simulink model "LQR_nonlinearized"  (R2019a)
settings: Solver=VariableStepAuto  StartTime=0.0  StopTime=10.0  RelTol=1e-3
values from neighbouring files (symbols this model uses):
  A = [0, 0, 1, 0 ... (first row only)    [LQR_v1.m]
  B = [0; 0; 0; b41]    [LQR_v1.m]
  C = [1, 0, 0, 0 ... (first row only)    [LQR_v1.m]
  g = 9.81    [LQR_v1.m]
  hb = 0.37    [LQR_v1.m]
  Igz = 0.061    [LQR_v1.m]
  Init_cond = [roll_angel, precession_angle, roll_rate, precession_rate]    [LQR_v1.m]
  init_precession_angle = 0    [LQR_v1.m]
  init_precession_rate = 0    [LQR_v1.m]
  init_roll_angle = 0.34    [LQR_v1.m]
  init_roll_rate = 0    [LQR_v1.m]
  K = lqr( A, B, Q, R )    [LQR_v1.m]
  k1 = 2*( Icx + Igx )    (= 0.141)    [LQR_v1.m]
  k2 = 2*( Icy + Igy )    (= 0.181)    [LQR_v1.m]
  k3 = 2*( Icz + Igz )    (= 0.322)    [LQR_v1.m]
  k4 = Ibx + 2*Igbx + 2*Isx    (= 10.2)    [LQR_v1.m]
  k5 = k1 - k3    (= -0.181)    [LQR_v1.m]
  k6 = hb*mb + 2*hg*(mg + mc + mgb) + 2*hs*ms    (= 26.27)    [LQR_v1.m]
  k7 = ( hb^2 )*mb + 2*( hg^2 )*( mg + mc + mgb ) + 2*( hs^2 )*ms    (= 9.7199)    [LQR_v1.m]
  omega = 532.6    [LQR_v1.m]
settings Model: Creator=daniel  LastModifiedBy=nata9
settings DataIOCC: ReturnWorkspaceOutputs=off
settings DebuggingCC: ArithmeticOperatorsInVariantConditions=warning
settings SFSimCC: SimUseLocalCustomCode=off
settings RTWCC: RTWUseLocalCustomCode=off

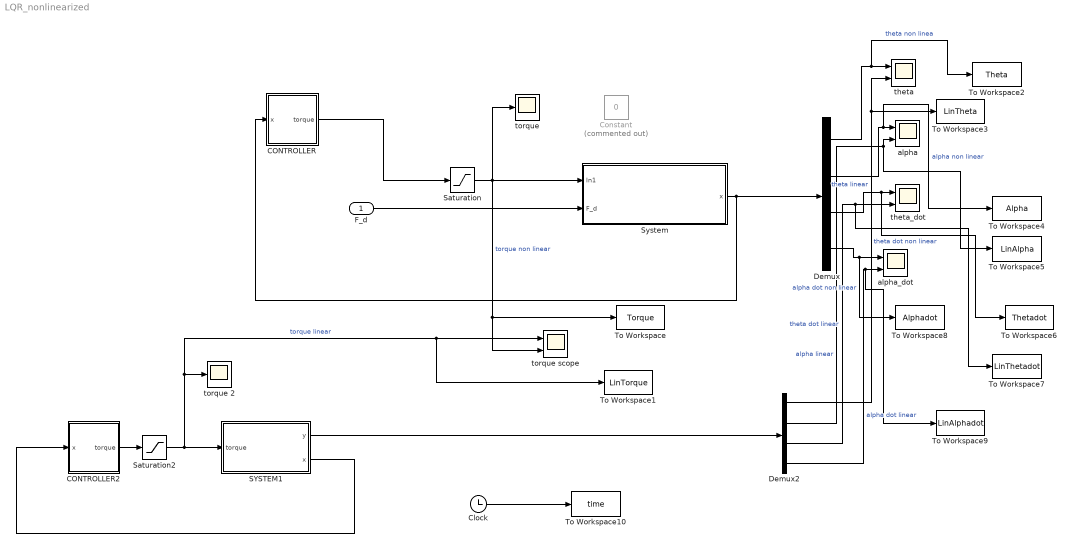
== system LQR_nonlinearized ==
  F_d : Inport
  " System" : Subsystem
  CONTROLLER : Subsystem
  CONTROLLER2 : Subsystem
  Clock : Clock
  Constant : Constant  Commented=on  Value=0
  Demux : Demux
  Demux2 : Demux
  SYSTEM1 : Subsystem
  Saturation : Saturate  UpperLimit=120  LowerLimit=-120
  Saturation2 : Saturate  UpperLimit=120  LowerLimit=-120
  To Workspace : ToWorkspace  VariableName=Torque  SampleTime=-1
  To Workspace1 : ToWorkspace  VariableName=LinTorque  SampleTime=-1
  To Workspace10 : ToWorkspace  VariableName=time  SampleTime=-1
  To Workspace2 : ToWorkspace  VariableName=Theta  SampleTime=-1
  To Workspace3 : ToWorkspace  VariableName=LinTheta  SampleTime=-1
  To Workspace4 : ToWorkspace  VariableName=Alpha  SampleTime=-1
  To Workspace5 : ToWorkspace  VariableName=LinAlpha  SampleTime=-1
  To Workspace6 : ToWorkspace  VariableName=Thetadot  SampleTime=-1
  To Workspace7 : ToWorkspace  VariableName=LinThetadot  SampleTime=-1
  To Workspace8 : ToWorkspace  VariableName=Alphadot  SampleTime=-1
  To Workspace9 : ToWorkspace  VariableName=LinAlphadot  SampleTime=-1
  alpha : Scope  NumInputPorts=2
  alpha_dot : Scope  NumInputPorts=2
  theta : Scope  NumInputPorts=2
  theta_dot : Scope  NumInputPorts=2
  "torque " : Scope
  torque 2 : Scope
  torque scope : Scope  NumInputPorts=2
  wires:
  CONTROLLER/1(torque) -> Saturation/1
  Saturation/1 -> "torque "/1, To Workspace/1, torque scope/2, " System"/1(In1)  "torque non linear"
  F_d/1 -> " System"/2(F_d)
  " System"/1(x) -> Demux/1, CONTROLLER/1("x ")
  Demux/1 -> To Workspace2/1, theta/1  "theta non linea"
  Demux/2 -> To Workspace4/1, alpha/1  "alpha non linear"
  Demux/3 -> To Workspace6/1, theta_dot/1  "theta dot non linear"
  Demux/4 -> To Workspace8/1, alpha_dot/1  "alpha dot non linear"
  Saturation2/1 -> torque 2/1, To Workspace1/1, torque scope/1, SYSTEM1/1("torque ")  "torque linear"
  CONTROLLER2/1(torque) -> Saturation2/1
  Demux2/1 -> theta/2, To Workspace3/1  "theta linear"
  SYSTEM1/1("y ") -> Demux2/1
  Demux2/2 -> To Workspace5/1, alpha/2  "alpha linear"
  SYSTEM1/2("x ") -> CONTROLLER2/1("x ")
  Demux2/4 -> To Workspace9/1, alpha_dot/2  "alpha dot linear"
  Demux2/3 -> To Workspace7/1, theta_dot/2  "theta dot linear"
  Clock/1 -> To Workspace10/1

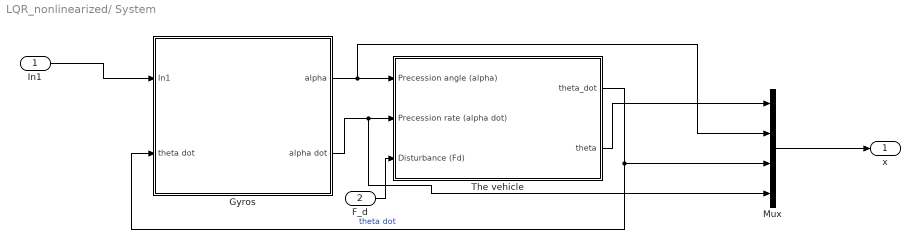
== system LQR_nonlinearized/ System ==
  In1 : Inport
  F_d : Inport  Port=2
  Gyros : Subsystem
  Mux : Mux
  The vehicle : Subsystem
  x : Outport
  wires:
  F_d/1 -> The vehicle/3(Disturbance (Fd))
  The vehicle/1(theta_dot) -> Mux/3, Gyros/2(theta dot)  "theta dot"
  Gyros/1(alpha) -> Mux/2, The vehicle/1("Precession angle (alpha) ")
  In1/1 -> Gyros/1(In1)
  Gyros/2(alpha dot) -> Mux/4, The vehicle/2(Precession rate (alpha dot))
  The vehicle/2(theta) -> Mux/1
  Mux/1 -> x/1

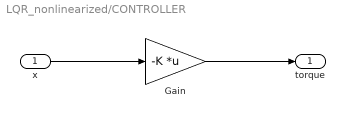
== system LQR_nonlinearized/CONTROLLER ==
  "x " : Inport
  "Gain " : Gain  Gain=-K  Multiplication=Matrix(K*u)
  torque : Outport
  wires:
  "Gain "/1 -> torque/1
  "x "/1 -> "Gain "/1

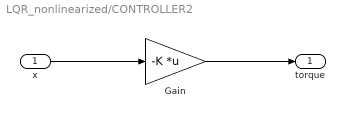
== system LQR_nonlinearized/CONTROLLER2 ==
  "x " : Inport
  "Gain " : Gain  Gain=-K  Multiplication=Matrix(K*u)
  torque : Outport
  wires:
  "Gain "/1 -> torque/1
  "x "/1 -> "Gain "/1

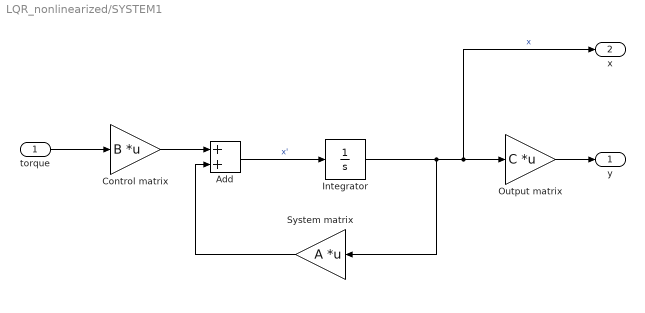
== system LQR_nonlinearized/SYSTEM1 ==
  "torque " : Inport
  Add : Sum
  Control matrix : Gain  Gain=B  Multiplication=Matrix(K*u)
  Integrator : Integrator  InitialCondition=Init_cond
  Output matrix : Gain  Gain=C  Multiplication=Matrix(K*u)
  System matrix : Gain  Gain=A  Multiplication=Matrix(K*u)
  "y " : Outport
  "x " : Outport  Port=2
  wires:
  Output matrix/1 -> "y "/1
  "torque "/1 -> Control matrix/1
  Integrator/1 -> "x "/1, Output matrix/1, System matrix/1  "x"
  Add/1 -> Integrator/1  "x'"
  Control matrix/1 -> Add/1
  System matrix/1 -> Add/2

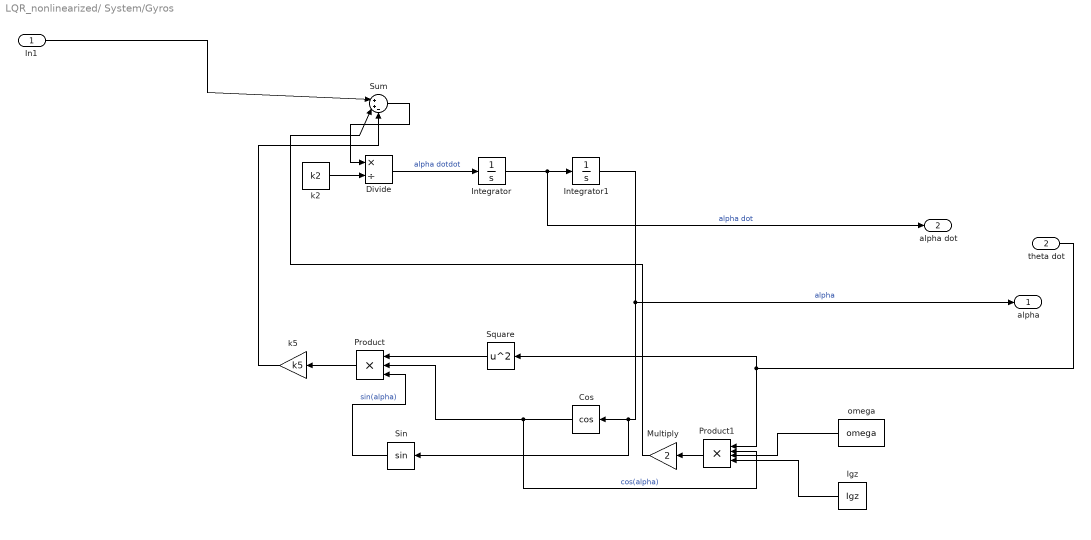
== system LQR_nonlinearized/ System/Gyros ==
  In1 : Inport
  theta dot : Inport  Port=2
  Cos : Trigonometry  Operator=cos
  Divide : Product  Inputs=*/
  Igz : Constant  Value=Igz
  Integrator : Integrator  InitialCondition=init_precession_rate
  Integrator1 : Integrator  InitialCondition=init_precession_angle
  Multiply : Gain  Gain=2
  Product : Product  Inputs=3
  Product1 : Product  Inputs=4
  Sin : Trigonometry
  Square : Math  Operator=square  SaturateOnIntegerOverflow=on
  Sum : Sum  Inputs=|++-
  k2 : Constant  Value=k2
  k5 : Gain  Gain=k5
  omega : Constant  Value=omega
  alpha : Outport
  alpha dot : Outport  Port=2
  wires:
  k5/1 -> Sum/3
  Igz/1 -> Product1/4
  Integrator/1 -> alpha dot/1, Integrator1/1  "alpha dot"
  omega/1 -> Product1/3
  Integrator1/1 -> alpha/1, Sin/1, Cos/1  "alpha"
  Divide/1 -> Integrator/1  "alpha dotdot"
  Multiply/1 -> Sum/2
  Cos/1 -> Product1/2, Product/2  "cos(alpha)"
  theta dot/1 -> Square/1, Product1/1
  k2/1 -> Divide/2
  Sum/1 -> Divide/1
  Square/1 -> Product/1
  Product1/1 -> Multiply/1
  Sin/1 -> Product/3  "sin(alpha)"
  Product/1 -> k5/1
  In1/1 -> Sum/1

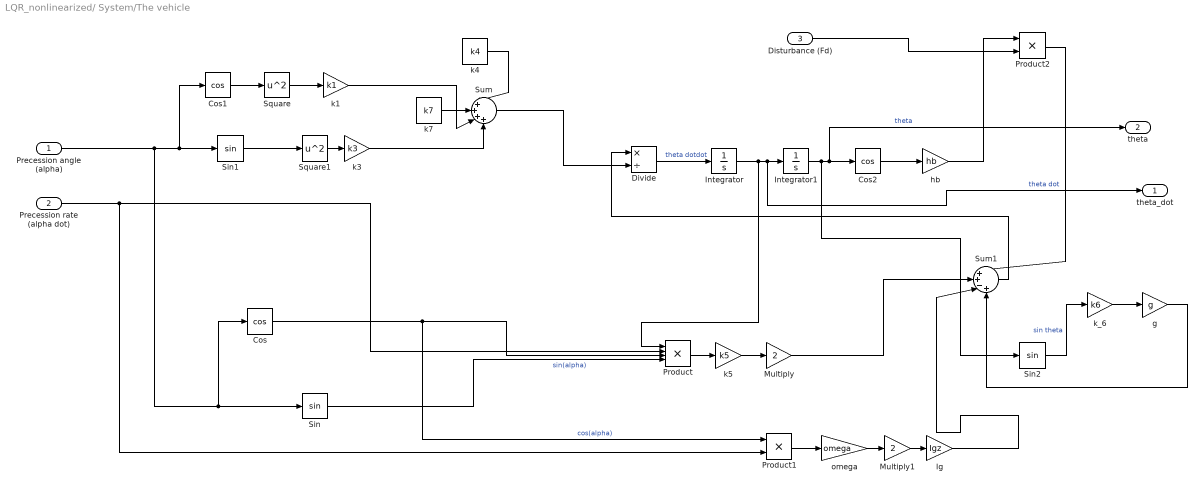
== system LQR_nonlinearized/ System/The vehicle ==
  "Precession angle (alpha) " : Inport
  Precession rate (alpha dot) : Inport  Port=2
  Disturbance (Fd) : Inport  Port=3
  Cos : Trigonometry  Operator=cos
  Cos1 : Trigonometry  Operator=cos
  Cos2 : Trigonometry  Operator=cos
  Divide : Product  Inputs=*/
  "Ig " : Gain  Gain=Igz
  Integrator : Integrator  InitialCondition=init_roll_rate
  Integrator1 : Integrator  InitialCondition=init_roll_angle
  Multiply : Gain  Gain=2
  Multiply1 : Gain  Gain=2
  Product : Product  Inputs=4
  Product1 : Product
  Product2 : Product
  Sin : Trigonometry
  Sin1 : Trigonometry
  Sin2 : Trigonometry
  Square : Math  Operator=square  SaturateOnIntegerOverflow=on
  Square1 : Math  Operator=square  SaturateOnIntegerOverflow=on
  Sum : Sum  Inputs=|++++
  Sum1 : Sum  Inputs=|++-+
  g : Gain  Gain=g
  "hb " : Gain  Gain=hb
  "k1 " : Gain  Gain=k1
  "k3 " : Gain  Gain=k3
  "k4 " : Constant  Value=k4
  "k5 " : Gain  Gain=k5
  "k7 " : Constant  Value=k7
  k_6 : Gain  Gain=k6
  "omega " : Gain  Gain=omega
  theta_dot : Outport
  theta : Outport  Port=2
  wires:
  "Precession angle (alpha) "/1 -> Sin/1, Cos/1, Cos1/1, Sin1/1
  "k3 "/1 -> Sum/4
  Sin2/1 -> k_6/1  "sin theta"
  Cos1/1 -> Square/1
  Sin1/1 -> Square1/1
  "hb "/1 -> Product2/1
  Product/1 -> "k5 "/1
  Disturbance (Fd)/1 -> Product2/2
  Cos2/1 -> "hb "/1
  Sin/1 -> Product/4  "sin(alpha)"
  "omega "/1 -> Multiply1/1
  Integrator1/1 -> Sin2/1, Cos2/1, theta/1  "theta"
  Cos/1 -> Product1/1, Product/3  "cos(alpha)"
  Integrator/1 -> Product/1, theta_dot/1, Integrator1/1  "theta dot"
  Square1/1 -> "k3 "/1
  "k7 "/1 -> Sum/2
  Divide/1 -> Integrator/1  "theta dotdot"
  Multiply/1 -> Sum1/2
  g/1 -> Sum1/4
  "k4 "/1 -> Sum/1
  Multiply1/1 -> "Ig "/1
  Precession rate (alpha dot)/1 -> Product1/2, Product/2
  "k1 "/1 -> Sum/3
  Sum/1 -> Divide/2
  Square/1 -> "k1 "/1
  "k5 "/1 -> Multiply/1
  Product1/1 -> "omega "/1
  k_6/1 -> g/1
  "Ig "/1 -> Sum1/3
  Product2/1 -> Sum1/1
  Sum1/1 -> Divide/1
